simulink model "BrakeController_Module"  (R2026a)
settings: Solver=VariableStepAuto
undefined symbols (not defined in the file): speed_tolerance
libraries: simulink x1
settings Model: Creator=Quang Huy  LastModifiedBy=ASUS

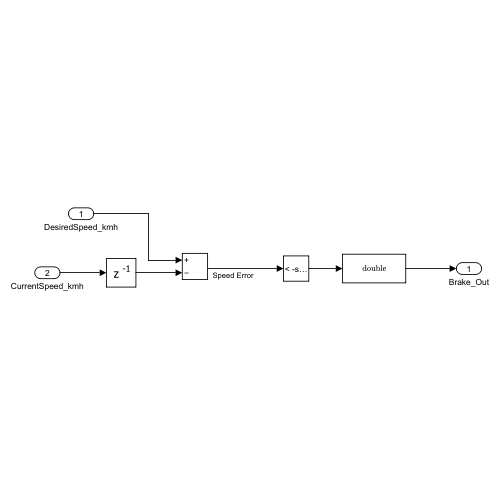
[thumbnail: Simulink's stored preview of the top-level diagram]
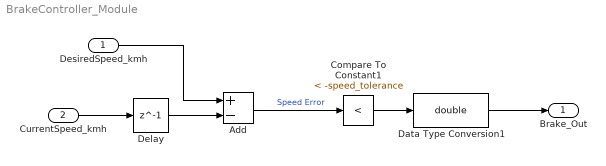
== system BrakeController_Module ==
  DesiredSpeed_kmh : Inport
  CurrentSpeed_kmh : Inport  Port=2
  Add : Sum  Inputs=+-
  Compare To Constant1 : simulink/Logic and Bit Operations/Compare To Constant  relop=<  const=-speed_tolerance  OutDataTypeStr=boolean
  Data Type Conversion1 : DataTypeConversion  OutDataTypeStr=double  SaturateOnIntegerOverflow=off  RndMeth=Floor
  Delay : Delay  DelayLength=1  InitialCondition=0  SampleTime=0.01
  Brake_Out : Outport
  wires:
  DesiredSpeed_kmh/1 -> Add/1
  CurrentSpeed_kmh/1 -> Delay/1
  Delay/1 -> Add/2
  Data Type Conversion1/1 -> Brake_Out/1
  Compare To Constant1/1 -> Data Type Conversion1/1
  Add/1 -> Compare To Constant1/1  "Speed Error"
